simulink model "Synthgas"  (R2025a)
settings: Solver=VariableStepAuto  StartTime=0.0  StopTime=3600  RelTol=1e-3
PreLoadFcn:
  | run('params_wte.m');
  | run('PEMElectrolysisSystemParameters.m');
  | run('params_co2el.m');
InitFcn:
  | run(fullfile(fileparts(bdroot),'params_wte.m'));
  | run(fullfile(fileparts(bdroot),'PEMElectrolysisSystemParameters.m'));
  | run(fullfile(fileparts(bdroot),'params_co2el.m'));
values from neighbouring files (symbols this model uses):
  A = [ -1/tauQ,        0 ... (first row only)    [params_wte.m]
  A_cm2 = 200    [params_co2el.m]
  alpha = wC * eta_burn * (44/12)    (= 1.43733333333)    [params_wte.m]
  B = [ (eta_th*LHV)/(1e6*tauQ) ... (first row only)    [params_wte.m]
  C = [0, 1]    [params_wte.m]
  D = 0    [params_wte.m]
  env_T = 20    [PEMElectrolysisSystemParameters.m]
  exchanger_air_area_fins = 2 * exchanger_N_fins * exchanger_W * exchanger_gap_H    (= 11.5625)    [PEMElectrolysisSystemParameters.m]
  exchanger_air_area_primary = 2 * (exchanger_N_tubes - 1) * exchanger_W * (exchanger_L + exchanger_gap_H)    (= 1.223125)    [PEMElectrolysisSystemParameters.m]
  exchanger_eta_fin = 0.7    [PEMElectrolysisSystemParameters.m]
  exchanger_N_tubes = 25    [PEMElectrolysisSystemParameters.m]
  exchanger_tube_H = 0.0015    [PEMElectrolysisSystemParameters.m]
  exchanger_W = 0.025    [PEMElectrolysisSystemParameters.m]
  F = 96485.33212    [params_co2el.m]
  gas_pipe_D = 0.01    [PEMElectrolysisSystemParameters.m]
  j_tab_mAcm2 = [0 ... (first row only)    [params_co2el.m]
  MW_CO = 28.0101e-3    (= 0.0280101)    [params_co2el.m]
  MW_CO2 = 44.0095e-3    (= 0.0440095)    [params_co2el.m]
  MW_H2 = 2.01588e-3    (= 0.00201588)    [params_co2el.m]
  N2_T = [-56.55, -50:10:-10, -5:1:5, 10:10:350]    [PEMElectrolysisSystemParameters.m]
  N_cell = 200    [params_co2el.m]
  p_bp = [0 ... (first row only)    [params_co2el.m]
  P_stack_max_W = p_max * (N_cell*A_cm2) / 1000    [params_co2el.m]
  stack_area = 280    [PEMElectrolysisSystemParameters.m]
  stack_mea_rho = 1800    [PEMElectrolysisSystemParameters.m]
  stack_num_cells = 50    [PEMElectrolysisSystemParameters.m]
  stack_num_channels = 8    [PEMElectrolysisSystemParameters.m]
  stack_t_gdl_A = 25    [PEMElectrolysisSystemParameters.m]
  stack_t_gdl_C = 250    [PEMElectrolysisSystemParameters.m]
  stack_t_membrane = 125    [PEMElectrolysisSystemParameters.m]
  stack_w_channels = 1    [PEMElectrolysisSystemParameters.m]
  V_tab = [0 ... (first row only)    [params_co2el.m]
  water_pipe_D = 0.01    [PEMElectrolysisSystemParameters.m]
undefined symbols (not defined in the file or in its folder): H2O, O2
libraries: fl_lib x48, nesl_utility x12, slpidlib x3
(part 3 of 3)

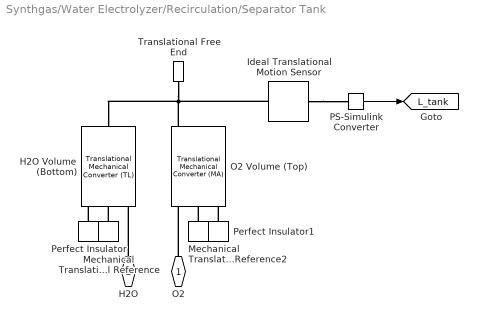
== system Synthgas/Water Electrolyzer/Recirculation/Separator Tank ==
  H2O Volume (Bottom) : fl_lib/Thermal Liquid/Elements/Translational Mechanical Converter (TL)  mech_orientation=foundation.enum.MechOrientationTranslational.Positive  displacement_spec=foundation.enum.DisplacementSpec.Calculate  x0=L_init m  interface_area=A m^2  dead_volume=A * 0.001 m^3  environment_spec=foundation.enum.pressure_spec.atmospheric  environment_pressure=0.101325 MPa  dynamic_compressibility=simscape.enum.onoff.off  p0=env_p MPa  T0=env_T degC  p_nominal=0.101325 MPa  T_nominal=293.15 K
      settings: InternalSimscapePortConfiguration="{\"Bottom\":[],\"Left\":[{\"id\":\"A\",\"label\":\"A\",\"type\":\"foundation.thermal_liquid.thermal_liquid\"},{\"id\":\"C\",\"label\":\"C\",\"type\":\"foundation.mechanical.translational.translational\"},{\"id\":\"H\",\"label\":\"H\",\"type\":\"foundation.thermal.thermal\"}],\"Right\":[{\"id\":\"R\",\"label\":\"R\",\"type\":\"foundation.mechanical.translational.translational\"}],\"Top\":[]}"
  Ideal Translational Motion Sensor : fl_lib/Mechanical/Mechanical Sensors/Ideal Translational Motion Sensor  reference=foundation.enum.MeasurementReference.absolute  acceleration_port=false  velocity_port=false  position_port=true  offset=L_init m
      settings: InternalSimscapePortConfiguration="{\"Bottom\":[],\"Left\":[{\"id\":\"R\",\"label\":\"R\",\"type\":\"foundation.mechanical.translational.translational\"}],\"Right\":[{\"id\":\"P\",\"label\":\"P\",\"type\":\"output\"}],\"Top\":[]}"
  Mechanical Translational Reference : fl_lib/Mechanical/Translational Elements/Mechanical Translational Reference
  Mechanical Translational Reference2 : fl_lib/Mechanical/Translational Elements/Mechanical Translational Reference
  O2 Volume (Top) : fl_lib/Moist Air/Elements/Translational Mechanical Converter (MA)  mech_orientation=foundation.enum.MechOrientationTranslational.Negative  displacement_spec=foundation.enum.DisplacementSpec.Calculate  length_init=L_init - L_max m  interface_area=A m^2  dead_volume=A * 0.001 m^3  area_A=pi*gas_pipe_D^2/4 m^2  pressure_spec=foundation.enum.pressure_spec.atmospheric  environment_pressure=0.101325 MPa  RH_ws=1  time_constant_cond=1e-3 s  time_constant_evap=1e-3 s  fraction_entrained=1  moisture_trace_gas_source=foundation.enum.moisture_trace_gas_source.none  moisture_source_spec=foundation.enum.MoistureSourceSpec.WaterVapor  vapor_from_liquid=false  moisture_mass_flow=0 kg/s  moisture_temperature_spec=foundation.enum.temperature_spec.atmospheric  moisture_temperature=293.15 K  trace_gas_mass_flow=0 kg/s  trace_gas_temperature_spec=foundation.enum.temperature_spec.atmospheric  trace_gas_temperature=293.15 K  p_init=env_p MPa  p_init_priority=foundation.enum.Priority.High  T_init=env_T degC  T_init_priority=foundation.enum.Priority.High  humidity_spec=foundation.enum.HumiditySpec.MoleFraction  RH_init=0  RH_init_priority=foundation.enum.Priority.None  x_w_init=0  x_w_init_priority=foundation.enum.Priority.None  y_w_init=0  y_w_init_priority=foundation.enum.Priority.High  HR_init=0  HR_init_priority=foundation.enum.Priority.None  Tw_init=287 K  Tw_init_priority=foundation.enum.Priority.High  trace_gas_spec=foundation.enum.trace_gas_spec.mole_fraction  x_g_init=1  x_g_init_priority=foundation.enum.Priority.None  y_g_init=1  y_g_init_priority=foundation.enum.Priority.High  r_d_init=0  r_d_init_priority=foundation.enum.Priority.High
      settings: InternalSimscapePortConfiguration="{\"Bottom\":[],\"Left\":[{\"id\":\"A\",\"label\":\"A\",\"type\":\"foundation.moist_air.moist_air\"},{\"id\":\"C\",\"label\":\"C\",\"type\":\"foundation.mechanical.translational.translational\"},{\"id\":\"H\",\"label\":\"H\",\"type\":\"foundation.thermal.thermal\"}],\"Right\":[{\"id\":\"R\",\"label\":\"R\",\"type\":\"foundation.mechanical.translational.translational\"},{\"id\":\"W\",\"label\":\"W\",\"type\":\"output\"},{\"id\":\"F\",\"label\":\"F\",\"type\":\"output\"}],\"Top\":[]}"
  PS-Simulink Converter : nesl_utility/PS-Simulink Converter  PhysicalDomain=network_engine_domain  SubClassName=ps_output  LeftPortType=input  RightPortType=output  PseudoPeriodic=off  Frequencies=[]  VectorFormat=inherit  Unit=m  AffineConversion=off
  Perfect Insulator : fl_lib/Thermal/Thermal Elements/Perfect Insulator  T_specify=off  T_priority=None  T=0 K  T_nominal_specify=off  T_nominal_value=1  T_nominal_unit=K
  Perfect Insulator1 : fl_lib/Thermal/Thermal Elements/Perfect Insulator  T_specify=off  T_priority=None  T=0 K  T_nominal_specify=off  T_nominal_value=1  T_nominal_unit=K
  Translational Free End : fl_lib/Mechanical/Translational Elements/Translational Free End  v_specify=off  v_priority=None  v=0 m/s  v_nominal_specify=off  v_nominal_value=1  v_nominal_unit=m/s
      settings: InternalSimscapePortConfiguration="{\"Bottom\":[],\"Left\":[{\"id\":\"V\",\"label\":\"\",\"type\":\"foundation.mechanical.translational.translational\"}],\"Right\":[],\"Top\":[]}"
  O2 : PMIOPort  Side=Left
  H2O : PMIOPort  Port=2  Side=Right
  tag scope: L_tank=global
  wires:
  PS-Simulink Converter/1 -> [L_tank]
  connections:
  Perfect Insulator/LConn1 -- H2O Volume (Bottom)/LConn3
  Mechanical Translational Reference/LConn1 -- H2O Volume (Bottom)/LConn2
  Ideal Translational Motion Sensor/RConn1 -- PS-Simulink Converter/LConn1
  Mechanical Translational Reference2/LConn1 -- O2 Volume (Top)/LConn2
  Perfect Insulator1/LConn1 -- O2 Volume (Top)/LConn3
  H2O/RConn1 -- H2O Volume (Bottom)/LConn1
  O2/RConn1 -- O2 Volume (Top)/LConn1
  Ideal Translational Motion Sensor/LConn1 -- H2O Volume (Bottom)/RConn1 -- Translational Free End/LConn1 -- O2 Volume (Top)/RConn1
